simulink model "Libreria"  (R2017a)
settings: Solver=VariableStepAuto  StartTime=0.0  StopTime=10.0  RelTol=1e-3
undefined symbols (not defined in the file or in its folder): st_time3
libraries: fl_lib x63, powerlib x30, nesl_utility x24, powerlib_meascontrol x9
(part 1 of 2)
settings Model: Creator=erich  LastModifiedBy=erich

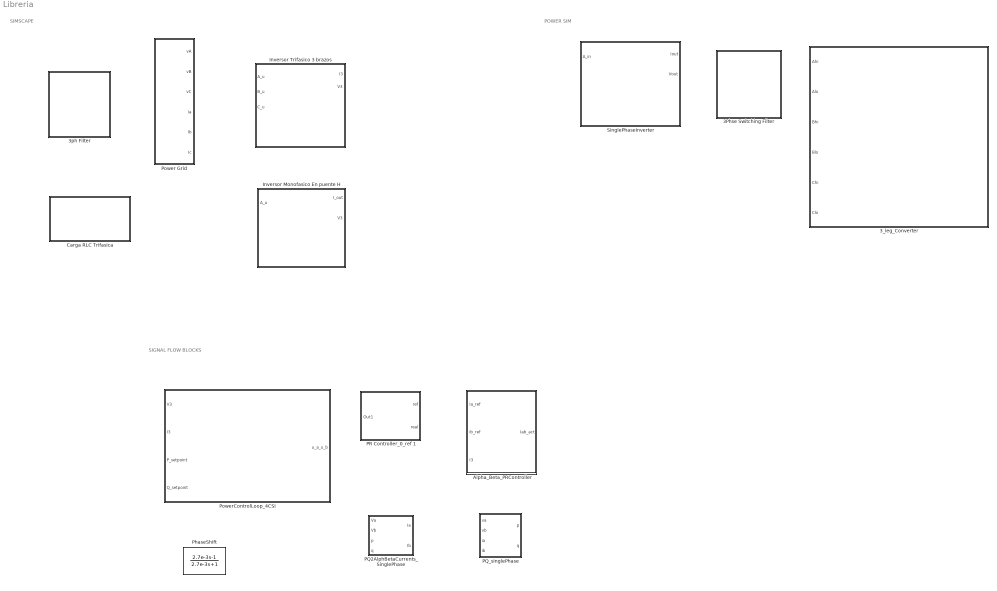
== system Libreria ==
  note: SIMSCAPE
  note: POWER SIM
  note: SIGNAL FLOW BLOCKS
  3Phse Switching Filter : Subsystem  mask{Lf=4e-3, rLf=1e-3, Cf=2.2e-6, rCf=1e-3}
      mask prompts: Lf "Inductancia (H)"; rLf "Resistencia parasita serie L (Ohm)"; Cf "Capacitancia (f)"; rCf "Resistencia parasita C serie"
      mask DialogControl DescTextVar Prompt: Configuracion del Filtro LC
      mask Display:
      | port_label('lconn', 1, 'A_{in}', 'texmode', 'on')
      | port_label('lconn', 2, 'B_{in}', 'texmode', 'on')
      | port_label('lconn', 3, 'B_{in}', 'texmode', 'on')
      | port_label('rconn', 1, 'A_{out}', 'texmode', 'on')
      | port_label('rconn', 2, 'B_{out}', 'texmode', 'on')
      | port_label('rconn', 3, 'C_{out}', 'texmode', 'on')
      | 
      | 
      | plot([.2 .5], [.7 .7])
      | plot([.5 .6], [.7 .3])
      | plot([.6 .7], [.3 .3])
      | 
      | text(.2, .8, '\fontsize{12} H(\omega)', 'texmode', 'on')
      | text(.6, .25, '\fontsize{12} \omega', 'texmode', 'on')
  3_leg_Converter : Subsystem
      mask Display:
      | port_label('input', 1, 'Ahi')
      | port_label('input', 2, 'Alo')
      | port_label('input', 3, 'Bhi')
      | port_label('input', 4, 'Blo')
      | port_label('input', 5, 'Chi')
      | port_label('input', 6, 'Clo')
      | 
      | port_label('rconn', 1, 'A')
      | port_label('rconn', 2, 'B')
      | port_label('rconn', 3, 'C')
      | port_label('rconn', 4, 'Collector')
      | port_label('rconn', 5, 'Emitter')
      | 
      | lvx = [.1 .1];
      | lvy = [.1 .2];
      | lhx = [.1 .2];
      | lhy = [.1 .1];
      | 
      | 
      | % se dibujan los interruptores de la izquierda
      | plot(lvx+.07, lvy*.8+.028+.1)
      | plot(lvx+.1, lvy+.1)
      | plot(lhx*.5+.15, lhy+.1)
      | plot(lhx*.5+.15, lhy+.2)
      | plot(lhx*.5+.07, lhy+.15)
      | 
      | d=0.5;
      | 
      | plot(lvx+.07, lvy*.8+.028+.1+d)
      | plot(lvx+.1, lvy+.1+d)
      | plot(lhx*.5+.15, lhy+.1+d)
      | plot(lhx*.5+.15, lhy+.2+d)
      | plot(lhx*.5+.07, lhy+.15+d)
      | 
      | 
      | % se dibujan los interruptores del medio
      | h=.3;
      | 
      | plot(lvx+.07+h, lvy*.8+.028+.1)
      | plot(lvx+.1+h, lvy+.1)
      | plot(lhx*.5+.15+h, lhy+.1)
      | plot(lhx*.5+.15+h, lhy+.2)
      | plot(lhx*.5+.07+h, lhy+.15)
      | 
      | plot(lvx+.07+h, lvy*.8+.028+.1+d)
      | plot(lvx+.1+h, lvy+.1+d)
      | plot(lhx*.5+.15+h, lhy+.1+d)
      | plot(lhx*.5+.15+h, lhy+.2+d)
      | plot(lhx*.5+.07+h, lhy+.15+d)
      | 
      | % se dibujan los interruptores de la derecha
      | h=.6
      | 
      | plot(lvx+.07+h, lvy*.8+.028+.1)
      | plot(lvx+.1+h, lvy+.1)
      | plot(lhx*.5+.15+h, lhy+.1)
      | plot(lhx*.5+.15+h, lhy+.2)
      | plot(lhx*.5+.07+h, lhy+.15)
      | 
      | plot(lvx+.07+h, lvy*.8+.028+.1+d)
      | plot(lvx+.1+h, lvy+.1+d)
      | plot(lhx*.5+.15+h, lhy+.1+d)
      | plot(lhx*.5+.15+h, lhy+.2+d)
      | plot(lhx*.5+.07+h, lhy+.15+d)
      | 
      | 
      | % se conectan los interruptores.
      | plot(lvx+.15, lvy*4-.1)
      | plot(lvx+.15+.3, lvy*4-.1)
      | plot(lvx+.15+.6, lvy*4-.1)
      | 
      | 
      | plot(lvx+.15, lvy+.7)
      | plot(lvx+.15+.3, lvy+.7)
      | plot(lvx+.15+.6, lvy+.7)
      | 
      | plot(lvx+.15, lvy)
      | plot(lvx+.15+.3, lvy)
      | plot(lvx+.15+.6, lvy)
      | 
      | plot(lhx*6-.35, lhy)
      | plot(lhx*6-.35, lhy+.8)
      | 
      | % raul esteban alzate 313 515 86 11
  3ph Filter : Subsystem
  Alpha_Beta_PRController : Subsystem
      mask Display:
      | port_label('input', 1, '\fontsize{13} \alpha_{ref}', 'texmode', 'on')
      | port_label('input', 2, '\fontsize{13} \beta_{ref}', 'texmode', 'on')
      | port_label('input', 3, '\fontsize{13} [ a, b, c ]', 'texmode', 'on')
      | 
      | port_label('output', 1, '\fontsize{13} [ u_{a}, u_{b}, u_{c} ]', 'texmode', 'on')
      | 
      | 
      | %plot([.4 .6],.05+[.5 .7])
      | %plot([.4 .6],.05+[.9 .7])
      | %plot([.4 .4],.05+[.9 .5])
      | 
      | text(.53,.2,'\fontsize{25} \int', 'texmode', 'on')
      | plot(.65+[0:.01:pi/10], .2+sin(40*[0:.01:pi/10])/13)
      | 
      | %text(.5,.8,'\fontsize{15} PR_{\alpha \beta}', 'texmode', 'on')
  Carga RLC Trifasica : Subsystem
      mask Display:
      | port_label('lconn', 1, 'GND')
      | 
      | port_label('rconn', 1, 'Z_1', 'texmode', 'on')
      | port_label('rconn', 2, 'Z_2', 'texmode', 'on')
      | port_label('rconn', 3, 'Z_3', 'texmode', 'on')
      | 
      | plot([.15 .25], [.4 .4])
      | plot([.15 .25], [.48 .48])
      | plot([.20 .20], [.48 .6])
      | plot([.20 .20], [.4 .28])
      | 
      | plot(.43+abs(sin(200*[.2:.001:.5]/(2*pi))/15), [.2:.001:.5]+.1)
      | plot([.438 .438], [.2 .3])
      | plot([.438 .438], [.6 .7])
      | 
      | 
      | plot([.67 .73], [.6 .6])
      | plot([.67 .73], [.3 .3])
      | 
      | plot([.7 .7], [.2 .3])
      | plot([.7 .7], [.6 .7])
      | 
      | plot([.67 .67], [.6 .3])
      | plot([.73 .73], [.6 .3])
  Inversor Monofasico En puente H : Subsystem
      mask Display:
      | port_label('input', 1, 'Mos IN')
      | 
      | port_label('lconn', 1, 'DC +')
      | port_label('lconn', 2, 'DC -')
      | 
      | 
      | port_label('rconn', 1, 'out +')
      | port_label('rconn', 2, 'out -')
      | 
      | 
      | port_label('output', 1, 'I_{out}', 'texmode', 'on')
      | port_label('output', 2, 'V_{out}', 'texmode', 'on')
      | 
      | plot([0.1 .9], [0.1 .9])
      | plot([0.2 .4], [.7 .7])
      | plot([0.2 .24], [.65 .65])
      | plot([0.28 .32], [.65 .65])
      | plot([0.36 .40], [.65 .65])
      | 
      | plot([.5:.01:.7], .25+sin(30*[.2:.01:.4])/10)
  Inversor Trifasico 3 brazos : Subsystem
      mask Display:
      | port_label('input', 1, 'A_u')
      | port_label('input', 2, 'B_u')
      | port_label('input', 3, 'C_u')
      | 
      | port_label('lconn', 1, 'DC +')
      | port_label('lconn', 2, 'DC -')
      | 
      | 
      | port_label('rconn', 1, 'A')
      | port_label('rconn', 2, 'B')
      | port_label('rconn', 3, 'C')
      | 
      | port_label('output', 1, 'I_{3\Phi}', 'texmode', 'on')
      | port_label('output', 2, 'V_{3\Phi}', 'texmode', 'on')
      | 
      | plot([0.1 .9], [0.1 .9])
      | plot([0.2 .4], [.7 .7])
      | plot([0.2 .24], [.65 .65])
      | plot([0.28 .32], [.65 .65])
      | plot([0.36 .40], [.65 .65])
      | 
      | plot([.5:.01:.7], .25+sin(30*[.2:.01:.4])/10)
  PQ2AlphBetaCurrents_SinglePhase : MATLAB Function  TreatAsAtomicUnit=on
  PQ_singlePhase : MATLAB Function  TreatAsAtomicUnit=on
  PR Controller_0_ref 1 : Subsystem  mask{Kp=2/100, Ki=10, wa=20, w0=60*2*pi, st_time=2e-3}
      mask prompts: Kp "Ganancia Proporcional"; Ki "Ganancia Integral"; wa "Ancho camapana resonancia"; w0 "Frecuencia Central"; st_time "Tiempo muerto (Start)"
      mask Display:
      | port_label('input',1,'ref')
      | port_label('input',2,'sens')
      | port_label('output',1,'out')
      | 
      | plot(.4+[0:.01:pi/10], .32+sin(40*[0:.01:pi/10])/13)
      | 
      | plot([.4 .6],.05+[.5 .7])
      | plot([.4 .6],.05+[.9 .7])
      | plot([.4 .4],.05+[.9 .5])
      | 
      | text(.27,.37,'\fontsize{25} \int', 'texmode', 'on')
  PhaseShift : TransferFcn  Numerator=[2.7e-3 -1]  Denominator=[2.7e-3 1]
  Power Grid : Subsystem
  PowerControlLoop_4CSI : Subsystem
      mask Display:
      | port_label('input', 1, '\fontsize{14} V_{abc}', 'texmode', 'on')
      | port_label('input', 2, '\fontsize{14} I_{abc}', 'texmode', 'on')
      | port_label('input', 3, '\fontsize{14} P_{set}', 'texmode', 'on')
      | port_label('input', 4, '\fontsize{14} Q_{set}', 'texmode', 'on')
      | port_label('output', 1, '\fontsize{14} u_{\alpha, \beta}', 'texmode', 'on')
      | 
      | 
      | disp('\fontsize{12} Power Control for 3\Phi CSI', 'texmode', 'on')
  SinglePhaseInverter : Subsystem  mask{st_time=2e-3, f_sw=10000}
      mask prompts: st_time "Tiempo muerto (Start)"; f_sw "Switching frequency"
      mask Display:
      | port_label('input', 1, 'd', 'texmode', 'on')
      | 
      | port_label('lconn', 1, 'DC +')
      | port_label('lconn', 2, 'DC -')
      | 
      | 
      | port_label('rconn', 1, 'V_{out+}')
      | port_label('rconn', 2, 'B_{out-}')
      | 
      | 
      | port_label('output', 1, 'I_{out}', 'texmode', 'on')
      | port_label('output', 2, 'V_{out}', 'texmode', 'on')
      | 
      | plot([0.1 .9], [0.1 .9])
      | plot([0.2 .4], [.7 .7])
      | plot([0.2 .24], [.65 .65])
      | plot([0.28 .32], [.65 .65])
      | plot([0.36 .40], [.65 .65])
      | 
      | plot([.5:.01:.7], .25+sin(30*[.2:.01:.4])/10)

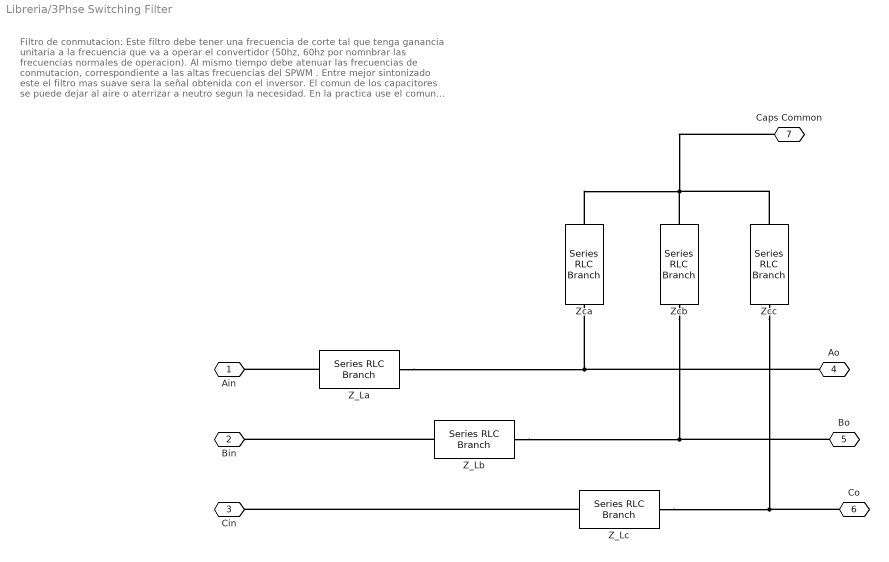
== system Libreria/3Phse Switching Filter ==
  note: Filtro de conmutacion:
      | Este filtro debe tener una frecuencia de corte tal
      | que tenga ganancia unitaria a la frecuencia que va
      | a operar el convertidor (50hz, 60hz por nomnbrar
      | las frecuencias normales de operacion). Al mismo
      | tiempo debe atenuar las frecuencias de conmutacion,
      | correspondiente a las altas frecuencias del SPWM .
      | Entre mejor sintonizado este el filtro mas suave sera
      | la señal obtenida con el inversor. El comun de los
      | capacitores se puede dejar al aire o aterrizar a neutro
      | segun la necesidad. En la practica use el comun al
      | aire para un inversor trifasico de verdad y dio buenos
      | resultados.
  Z_La : powerlib/Elements/Series RLC Branch  LConnTagsString=__new0  RConnTagsString=__new0  BranchType=RL  Resistance=rLf  Inductance=Lf  SetiL0=off  InitialCurrent=0  Capacitance=2.2e-6  Setx0=off  InitialVoltage=0  Measurements=None
  Z_Lb : powerlib/Elements/Series RLC Branch  LConnTagsString=__new0  RConnTagsString=__new0  BranchType=RL  Resistance=rLf  Inductance=Lf  SetiL0=off  InitialCurrent=0  Capacitance=2.2e-6  Setx0=off  InitialVoltage=0  Measurements=None
  Z_Lc : powerlib/Elements/Series RLC Branch  LConnTagsString=__new0  RConnTagsString=__new0  BranchType=RL  Resistance=rLf  Inductance=Lf  SetiL0=off  InitialCurrent=0  Capacitance=2.2e-6  Setx0=off  InitialVoltage=0  Measurements=None
  Zca : powerlib/Elements/Series RLC Branch  LConnTagsString=__new0  RConnTagsString=__new0  BranchType=RC  Resistance=rCf  Inductance=1e-9  SetiL0=off  InitialCurrent=0  Capacitance=Cf  Setx0=off  InitialVoltage=0  Measurements=None
  Zcb : powerlib/Elements/Series RLC Branch  LConnTagsString=__new0  RConnTagsString=__new0  BranchType=RC  Resistance=rCf  Inductance=1e-9  SetiL0=off  InitialCurrent=0  Capacitance=Cf  Setx0=off  InitialVoltage=0  Measurements=None
  Zcc : powerlib/Elements/Series RLC Branch  LConnTagsString=__new0  RConnTagsString=__new0  BranchType=RC  Resistance=rCf  Inductance=1e-9  SetiL0=off  InitialCurrent=0  Capacitance=Cf  Setx0=off  InitialVoltage=0  Measurements=None
  Ain : PMIOPort  Port=1  Side=Left
  Bin : PMIOPort  Port=2  Side=Left
  Cin : PMIOPort  Port=3  Side=Left
  Ao : PMIOPort  Port=4  Side=Right
  Bo : PMIOPort  Port=5  Side=Right
  Co : PMIOPort  Port=6  Side=Right
  Caps Common : PMIOPort  Port=7  Side=Right
  connections:
  Zcc/RConn1 -- Zcb/RConn1 -- Zca/RConn1 -- Caps Common/RConn1
  Z_Lb/RConn1 -- Bo/RConn1 -- Zcb/LConn1
  Z_Lc/RConn1 -- Co/RConn1 -- Zcc/LConn1
  Ao/RConn1 -- Z_La/RConn1 -- Zca/LConn1
  Z_La/LConn1 -- Ain/RConn1
  Z_Lb/LConn1 -- Bin/RConn1
  Z_Lc/LConn1 -- Cin/RConn1

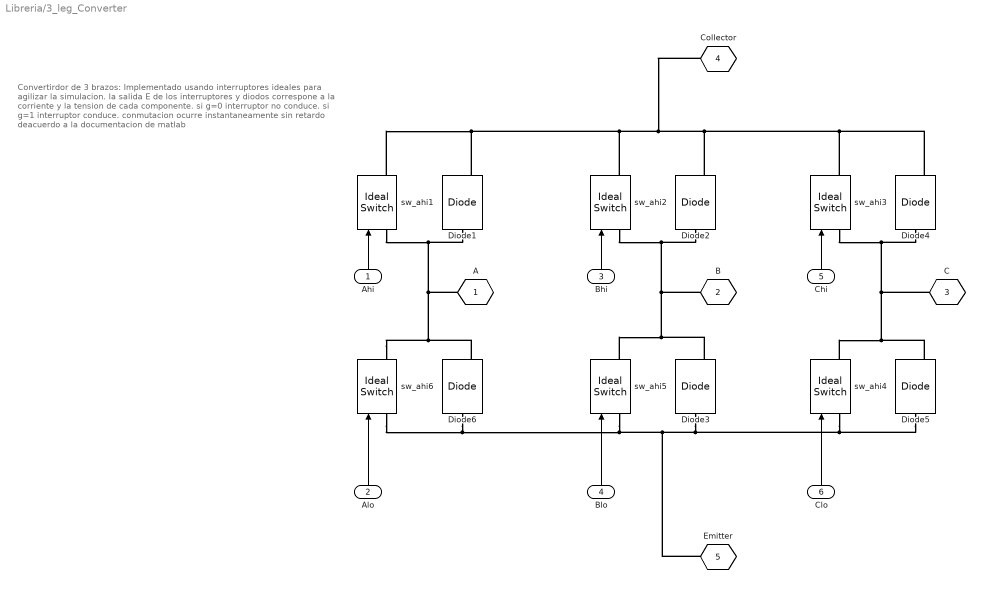
== system Libreria/3_leg_Converter ==
  note: Convertirdor de 3 brazos:
      |
      | Implementado usando interruptores
      | ideales para agilizar la simulacion.
      | la salida E de los interruptores y diodos correspone
      | a la corriente y la tension de cada componente.
      |
      | si g=0 interruptor no conduce.
      | si g=1 interruptor conduce.
      |
      | conmutacion ocurre instantaneamente sin
      | retardo deacuerdo a la documentacion de matlab
  Ahi : Inport
  Alo : Inport  Port=2
  Bhi : Inport  Port=3
  Blo : Inport  Port=4
  Chi : Inport  Port=5
  Clo : Inport  Port=6
   sw_ahi{1..6} (6 alike) : powerlib/Power Electronics/Ideal Switch  Ron=20e-3  Lon=0  IC=0  Rs=1e6  Cs=10e-12  Measurements=on
  Diode{1..6} (6 alike) : powerlib/Power Electronics/Diode  Ron=.2  Lon=0  Vf=0.8  IC=0  UseSnubber=0  Rs=0  Cs=0  Measurements=on
  " A" : PMIOPort  Tag=PMCPort  Port=1  Side=Right
  B : PMIOPort  Tag=PMCPort  Port=2  Side=Right
  C : PMIOPort  Tag=PMCPort  Port=3  Side=Right
  Collector : PMIOPort  Tag=PMCPort  Port=4  Side=Right
  Emitter : PMIOPort  Tag=PMCPort  Port=5  Side=Right
  wires:
  Clo/1 -> " sw_ahi4"/1
  Alo/1 -> " sw_ahi6"/1
  Ahi/1 -> " sw_ahi1"/1
  Blo/1 -> " sw_ahi5"/1
  Bhi/1 -> " sw_ahi2"/1
  Chi/1 -> " sw_ahi3"/1
  connections:
  Diode3/RConn1 -- " sw_ahi5"/RConn1 -- B/RConn1 -- " sw_ahi2"/LConn1 -- Diode2/LConn1
  Diode3/LConn1 -- " sw_ahi4"/LConn1 -- Diode5/LConn1 -- Emitter/RConn1 -- " sw_ahi5"/LConn1 -- Diode6/LConn1 -- " sw_ahi6"/LConn1
  Diode2/RConn1 -- " sw_ahi3"/RConn1 -- Diode4/RConn1 -- Collector/RConn1 -- " sw_ahi2"/RConn1 -- " sw_ahi1"/RConn1 -- Diode1/RConn1
  " sw_ahi6"/RConn1 -- Diode6/RConn1 -- " A"/RConn1 -- " sw_ahi1"/LConn1 -- Diode1/LConn1
  " sw_ahi4"/RConn1 -- Diode5/RConn1 -- C/RConn1 -- " sw_ahi3"/LConn1 -- Diode4/LConn1

== system Libreria/3ph Filter ==
  CdcS1 : fl_lib/Electrical/Electrical Elements/Capacitor  c=3.5 uF  r=1e-6 Ohm  g=0 1/Ohm  i_specify=off  i_priority=None  i=0 A  i_nominal_specify=off  i_nominal_unit=A  i_nominal_value=1  v_specify=off  v_priority=None  v=0 V  v_nominal_specify=off  v_nominal_unit=V  v_nominal_value=1  vc_specify=on  vc_priority=High  vc=0 V  vc_nominal_specify=off  vc_nominal_unit=V  vc_nominal_value=1
  CdcS2 : fl_lib/Electrical/Electrical Elements/Capacitor  c=3.5 uF  r=1e-6 Ohm  g=0 1/Ohm  i_specify=off  i_priority=None  i=0 A  i_nominal_specify=off  i_nominal_unit=A  i_nominal_value=1  v_specify=off  v_priority=None  v=0 V  v_nominal_specify=off  v_nominal_unit=V  v_nominal_value=1  vc_specify=on  vc_priority=High  vc=0 V  vc_nominal_specify=off  vc_nominal_unit=V  vc_nominal_value=1
  CdcS3 : fl_lib/Electrical/Electrical Elements/Capacitor  c=3.5 uF  r=1e-6 Ohm  g=0 1/Ohm  i_specify=off  i_priority=None  i=0 A  i_nominal_specify=off  i_nominal_unit=A  i_nominal_value=1  v_specify=off  v_priority=None  v=0 V  v_nominal_specify=off  v_nominal_unit=V  v_nominal_value=1  vc_specify=on  vc_priority=High  vc=0 V  vc_nominal_specify=off  vc_nominal_unit=V  vc_nominal_value=1
  LA_filt : fl_lib/Electrical/Electrical Elements/Inductor  l=6.2 mH  r=0.1 Ohm  g=1e-6 1/Ohm  i_specify=off  i_priority=None  i=0 A  i_nominal_specify=off  i_nominal_unit=A  i_nominal_value=1  v_specify=off  v_priority=None  v=0 V  v_nominal_specify=off  v_nominal_unit=V  v_nominal_value=1  i_L_specify=on  i_L_priority=High  i_L=0 A  i_L_nominal_specify=off  i_L_nominal_unit=A  i_L_nominal_value=1
  LB_filt : fl_lib/Electrical/Electrical Elements/Inductor  l=6.2 mH  r=2 Ohm  g=1e-6 1/Ohm  i_specify=off  i_priority=None  i=0 A  i_nominal_specify=off  i_nominal_unit=A  i_nominal_value=1  v_specify=off  v_priority=None  v=0 V  v_nominal_specify=off  v_nominal_unit=V  v_nominal_value=1  i_L_specify=on  i_L_priority=High  i_L=0 A  i_L_nominal_specify=off  i_L_nominal_unit=A  i_L_nominal_value=1
  LC_filt : fl_lib/Electrical/Electrical Elements/Inductor  l=6.2 mH  r=2 Ohm  g=1e-6 1/Ohm  i_specify=off  i_priority=None  i=0 A  i_nominal_specify=off  i_nominal_unit=A  i_nominal_value=1  v_specify=off  v_priority=None  v=0 V  v_nominal_specify=off  v_nominal_unit=V  v_nominal_value=1  i_L_specify=on  i_L_priority=High  i_L=0 A  i_L_nominal_specify=off  i_L_nominal_unit=A  i_L_nominal_value=1
  Ain : PMIOPort  Port=1  Side=Left
  Aout : PMIOPort  Port=2  Side=Right
  Bin : PMIOPort  Port=3  Side=Left
  Bout : PMIOPort  Port=4  Side=Right
  Cin : PMIOPort  Port=5  Side=Left
  Cout : PMIOPort  Port=6  Side=Right
  connections:
  CdcS1/RConn1 -- Aout/RConn1 -- LA_filt/RConn1
  CdcS2/LConn1 -- CdcS1/LConn1 -- CdcS3/LConn1
  CdcS3/RConn1 -- Bout/RConn1 -- LB_filt/RConn1
  CdcS2/RConn1 -- Cout/RConn1 -- LC_filt/RConn1
  LC_filt/LConn1 -- Cin/RConn1
  LA_filt/LConn1 -- Ain/RConn1
  LB_filt/LConn1 -- Bin/RConn1

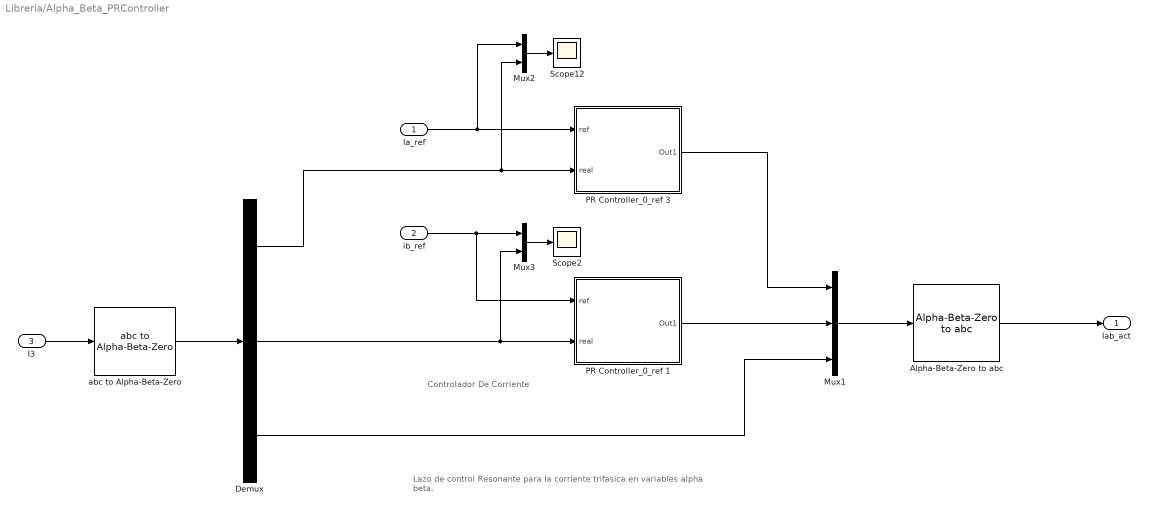
== system Libreria/Alpha_Beta_PRController ==
  note: Controlador De Corriente
  note: Lazo de control Resonante para la
      | corriente trifasica en variables alpha beta.
  Ia_ref : Inport
  ib_ref : Inport  Port=2
  I3 : Inport  Port=3
  Alpha-Beta-Zero to abc : powerlib_meascontrol/Transformations/Alpha-Beta-Zero to abc
      settings: SourceProductName=Simscape Power Systems  SourceProductBaseCode=PS
  Demux : Demux  Outputs=3
  Mux1 : Mux  Inputs=3
  Mux2 : Mux  Inputs=2
  Mux3 : Mux  Inputs=2
  PR Controller_0_ref 1 : Subsystem
      mask Display:
      | port_label('input',1,'ref')
      | port_label('input',2,'sens')
      | port_label('output',1,'out')
      | 
      | plot(.4+[0:.01:pi/10], .32+sin(40*[0:.01:pi/10])/13)
      | 
      | plot([.4 .6],.05+[.5 .7])
      | plot([.4 .6],.05+[.9 .7])
      | plot([.4 .4],.05+[.9 .5])
      | 
      | text(.27,.37,'\fontsize{25} \int', 'texmode', 'on')
  PR Controller_0_ref 3 : Subsystem
      mask Display:
      | port_label('input',1,'ref')
      | port_label('input',2,'sens')
      | port_label('output',1,'out')
      | 
      | plot(.4+[0:.01:pi/10], .32+sin(40*[0:.01:pi/10])/13)
      | 
      | plot([.4 .6],.05+[.5 .7])
      | plot([.4 .6],.05+[.9 .7])
      | plot([.4 .4],.05+[.9 .5])
      | 
      | text(.27,.37,'\fontsize{25} \int', 'texmode', 'on')
  Scope12 : Scope
  Scope2 : Scope
  abc to Alpha-Beta-Zero : powerlib_meascontrol/Transformations/abc to Alpha-Beta-Zero
      settings: SourceProductName=Simscape Power Systems
  Iab_act : Outport
  wires:
  I3/1 -> abc to Alpha-Beta-Zero/1
  Mux2/1 -> Scope12/1
  Demux/2 -> PR Controller_0_ref 1/2(real), Mux3/2
  PR Controller_0_ref 1/1(Out1) -> Mux1/2
  Mux1/1 -> Alpha-Beta-Zero to abc/1
  Mux3/1 -> Scope2/1
  Alpha-Beta-Zero to abc/1 -> Iab_act/1
  abc to Alpha-Beta-Zero/1 -> Demux/1
  ib_ref/1 -> PR Controller_0_ref 1/1(ref), Mux3/1
  Ia_ref/1 -> Mux2/1, PR Controller_0_ref 3/1(ref)
  PR Controller_0_ref 3/1(Out1) -> Mux1/1
  Demux/3 -> Mux1/3
  Demux/1 -> Mux2/2, PR Controller_0_ref 3/2(real)

== system Libreria/Carga RLC Trifasica ==
  Capacitor : fl_lib/Electrical/Electrical Elements/Capacitor  c=100e-6 uF  r=1e-6 Ohm  g=0 1/Ohm  i_specify=off  i_priority=None  i=0 A  i_nominal_specify=off  i_nominal_unit=A  i_nominal_value=1  v_specify=off  v_priority=None  v=0 V  v_nominal_specify=off  v_nominal_unit=V  v_nominal_value=1  vc_specify=off  vc_priority=High  vc=0 V  vc_nominal_specify=off  vc_nominal_unit=V  vc_nominal_value=1
  Capacitor1 : fl_lib/Electrical/Electrical Elements/Capacitor  c=100e-6 uF  r=1e-6 Ohm  g=0 1/Ohm  i_specify=off  i_priority=None  i=0 A  i_nominal_specify=off  i_nominal_unit=A  i_nominal_value=1  v_specify=off  v_priority=None  v=0 V  v_nominal_specify=off  v_nominal_unit=V  v_nominal_value=1  vc_specify=off  vc_priority=High  vc=0 V  vc_nominal_specify=off  vc_nominal_unit=V  vc_nominal_value=1
  Capacitor2 : fl_lib/Electrical/Electrical Elements/Capacitor  c=100e-6 uF  r=1e-6 Ohm  g=0 1/Ohm  i_specify=off  i_priority=None  i=0 A  i_nominal_specify=off  i_nominal_unit=A  i_nominal_value=1  v_specify=off  v_priority=None  v=0 V  v_nominal_specify=off  v_nominal_unit=V  v_nominal_value=1  vc_specify=off  vc_priority=High  vc=0 V  vc_nominal_specify=off  vc_nominal_unit=V  vc_nominal_value=1
  Inductor : fl_lib/Electrical/Electrical Elements/Inductor  l=5200 mH  r=0 Ohm  g=100e-9 1/Ohm  i_specify=off  i_priority=None  i=0 A  i_nominal_specify=off  i_nominal_unit=A  i_nominal_value=1  v_specify=off  v_priority=None  v=0 V  v_nominal_specify=off  v_nominal_unit=V  v_nominal_value=1  i_L_specify=off  i_L_priority=High  i_L=0 A  i_L_nominal_specify=off  i_L_nominal_unit=A  i_L_nominal_value=1
  Inductor1 : fl_lib/Electrical/Electrical Elements/Inductor  l=5200 mH  r=0 Ohm  g=100e-9 1/Ohm  i_specify=off  i_priority=None  i=0 A  i_nominal_specify=off  i_nominal_unit=A  i_nominal_value=1  v_specify=off  v_priority=None  v=0 V  v_nominal_specify=off  v_nominal_unit=V  v_nominal_value=1  i_L_specify=off  i_L_priority=High  i_L=0 A  i_L_nominal_specify=off  i_L_nominal_unit=A  i_L_nominal_value=1
  Inductor2 : fl_lib/Electrical/Electrical Elements/Inductor  l=5200 mH  r=0 Ohm  g=100e-9 1/Ohm  i_specify=off  i_priority=None  i=0 A  i_nominal_specify=off  i_nominal_unit=A  i_nominal_value=1  v_specify=off  v_priority=None  v=0 V  v_nominal_specify=off  v_nominal_unit=V  v_nominal_value=1  i_L_specify=off  i_L_priority=High  i_L=0 A  i_L_nominal_specify=off  i_L_nominal_unit=A  i_L_nominal_value=1
  RLA : fl_lib/Electrical/Electrical Elements/Resistor  R=15 Ohm  i_specify=off  i_priority=None  i=0 A  i_nominal_specify=off  i_nominal_unit=A  i_nominal_value=1  v_specify=off  v_priority=None  v=0 V  v_nominal_specify=off  v_nominal_unit=V  v_nominal_value=1
  RLB : fl_lib/Electrical/Electrical Elements/Resistor  R=15 Ohm  i_specify=off  i_priority=None  i=0 A  i_nominal_specify=off  i_nominal_unit=A  i_nominal_value=1  v_specify=off  v_priority=None  v=0 V  v_nominal_specify=off  v_nominal_unit=V  v_nominal_value=1
  RLC : fl_lib/Electrical/Electrical Elements/Resistor  R=15 Ohm  i_specify=off  i_priority=None  i=0 A  i_nominal_specify=off  i_nominal_unit=A  i_nominal_value=1  v_specify=off  v_priority=None  v=0 V  v_nominal_specify=off  v_nominal_unit=V  v_nominal_value=1
  Conn1 : PMIOPort  Port=1  Side=Right
  Conn2 : PMIOPort  Port=2  Side=Right
  Conn3 : PMIOPort  Port=3  Side=Right
  Conn4 : PMIOPort  Port=4  Side=Left
  connections:
  RLB/RConn1 -- Capacitor1/RConn1 -- Inductor1/RConn1 -- Conn4/RConn1 -- Inductor2/RConn1 -- Capacitor/RConn1 -- RLA/RConn1 -- Capacitor2/RConn1 -- Inductor/RConn1 -- RLC/RConn1
  RLA/LConn1 -- Inductor2/LConn1 -- Conn1/RConn1 -- Capacitor/LConn1
  RLC/LConn1 -- Capacitor2/LConn1 -- Conn3/RConn1 -- Inductor/LConn1
  RLB/LConn1 -- Conn2/RConn1 -- Capacitor1/LConn1 -- Inductor1/LConn1

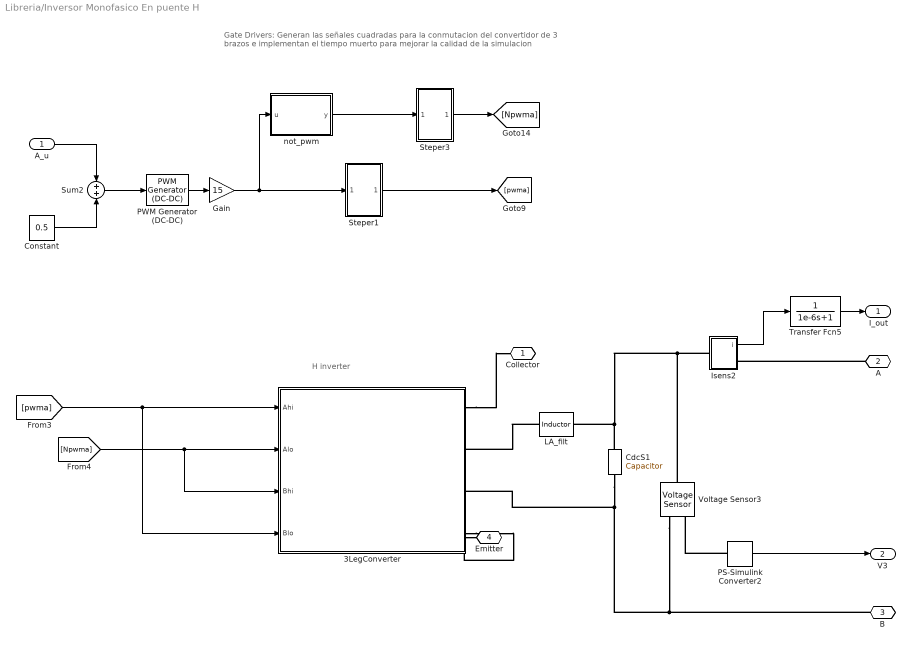
== system Libreria/Inversor Monofasico En puente H ==
  note: Gate Drivers: Generan las señales cuadradas para
      | la conmutacion del convertidor de 3 brazos e implementan el
      | tiempo muerto para mejorar la calidad de la simulacion
  note: H inverter
  A_u : Inport
  3LegConverter : Subsystem
      mask Display:
      | % entradas de conmutacion del mosfet
      | port_label('input',1,'Ahi')
      | port_label('input',2,'Alo')
      | port_label('input',3,'Bhi')
      | port_label('input',4,'Blo')
      | 
      | 
      | % puertos de conexion del inversor
      | port_label('rconn',1,'Collector') % + fuente dc
      | port_label('rconn',2,'Out +') % fase A
      | port_label('rconn',3,'Out -') % fase B
      | port_label('rconn',4,'Emitter') % ref fuente dc
      | 
      | 
      | plot([.4 .4],[.35 .7])
      | plot([.2 .4],[.52 .52])
      | plot([.46 .46],[.22 .85])
      | plot([.46 .7],[.73 .73])
      | plot([.46 .7],[.32 .32])
  CdcS1 : fl_lib/Electrical/Electrical Elements/Capacitor  c=3.5 uF  r=1e-6 Ohm  g=0 1/Ohm  i_specify=off  i_priority=None  i=0 A  i_nominal_specify=off  i_nominal_unit=A  i_nominal_value=1  v_specify=off  v_priority=None  v=0 V  v_nominal_specify=off  v_nominal_unit=V  v_nominal_value=1  vc_specify=on  vc_priority=High  vc=0 V  vc_nominal_specify=off  vc_nominal_unit=V  vc_nominal_value=1
  Constant : Constant  Value=0.5
  Gain : Gain  Gain=15
  Isens2 : Subsystem
  LA_filt : fl_lib/Electrical/Electrical Elements/Inductor  l=6.2 mH  r=0.1 Ohm  g=1e-6 1/Ohm  i_specify=off  i_priority=None  i=0 A  i_nominal_specify=off  i_nominal_unit=A  i_nominal_value=1  v_specify=off  v_priority=None  v=0 V  v_nominal_specify=off  v_nominal_unit=V  v_nominal_value=1  i_L_specify=on  i_L_priority=High  i_L=0 A  i_L_nominal_specify=off  i_L_nominal_unit=A  i_L_nominal_value=1
  PS-Simulink Converter2 : nesl_utility/PS-Simulink Converter  PhysicalDomain=network_engine_domain  SubClassName=ps_output  LeftPortType=input  RightPortType=output  PseudoPeriodic=off  Frequencies=[]  Unit=1  AffineConversion=off
  PWM Generator (DC-DC) : powerlib_meascontrol/Pulse & Signal Generators/PWM Generator (DC-DC)  Fsw=5000  Ts=0
  Steper1 : Subsystem
  Steper3 : Subsystem
  Sum2 : Sum
  Transfer Fcn5 : TransferFcn  Denominator=[1e-6 1]
  Voltage Sensor3 : fl_lib/Electrical/Electrical Sensors/Voltage Sensor
  not_pwm : MATLAB Function  TreatAsAtomicUnit=on
  Collector : PMIOPort  Port=1  Side=Left
  A : PMIOPort  Port=2  Side=Right
  B : PMIOPort  Port=3  Side=Right
  Emitter : PMIOPort  Port=4  Side=Left
  I_out : Outport
  V3 : Outport  Port=2
  wires:
  [pwma] -> 3LegConverter/4(Blo), 3LegConverter/1(Ahi)
  [Npwma] -> 3LegConverter/3(Bhi), 3LegConverter/2(Alo)
  Gain/1 -> Steper1/1(In1), not_pwm/1(u)
  Steper3/1(Out1) -> [Npwma]
  Constant/1 -> Sum2/2
  Sum2/1 -> PWM Generator (DC-DC)/1
  not_pwm/1(y) -> Steper3/1(In1)
  PWM Generator (DC-DC)/1 -> Gain/1
  Steper1/1(Out1) -> [pwma]
  A_u/1 -> Sum2/1
  Isens2/1(i) -> Transfer Fcn5/1
  PS-Simulink Converter2/1 -> V3/1
  Transfer Fcn5/1 -> I_out/1
  connections:
  3LegConverter/RConn4 -- Emitter/RConn1
  3LegConverter/RConn1 -- Collector/RConn1
  A/RConn1 -- Isens2/RConn1
  PS-Simulink Converter2/LConn1 -- Voltage Sensor3/RConn1
  CdcS1/RConn1 -- Isens2/LConn1 -- Voltage Sensor3/LConn1 -- LA_filt/RConn1
  LA_filt/LConn1 -- 3LegConverter/RConn2
  CdcS1/LConn1 -- B/RConn1 -- Voltage Sensor3/RConn2 -- 3LegConverter/RConn3

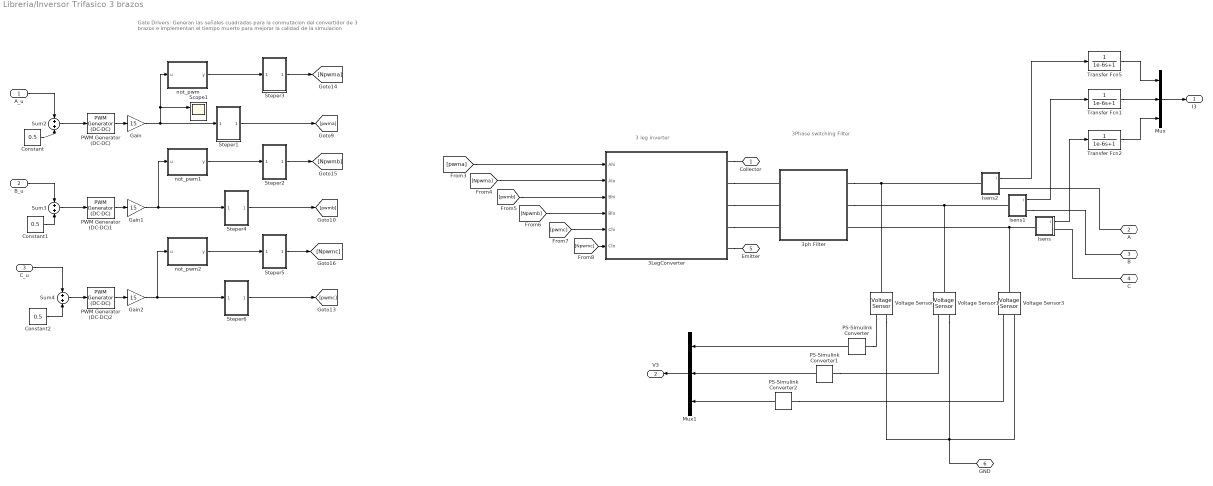
== system Libreria/Inversor Trifasico 3 brazos ==
  note: Gate Drivers: Generan las señales cuadradas para
      | la conmutacion del convertidor de 3 brazos e implementan el
      | tiempo muerto para mejorar la calidad de la simulacion
  note: 3 leg inverter
  note: 3Phase
      | switching
      | Filter
  A_u : Inport
  B_u : Inport  Port=2
  C_u : Inport  Port=3
  3LegConverter : Subsystem
      mask Display:
      | % entradas de conmutacion del mosfet
      | port_label('input',1,'Ahi')
      | port_label('input',2,'Alo')
      | port_label('input',3,'Bhi')
      | port_label('input',4,'Blo')
      | port_label('input',5,'Chi')
      | port_label('input',6,'Clo')
      | 
      | % puertos de conexion del inversor
      | port_label('rconn',1,'Collector') % + fuente dc
      | port_label('rconn',2,'A') % fase A
      | port_label('rconn',3,'B') % fase B
      | port_label('rconn',4,'C') % fase C
      | port_label('rconn',5,'Emitter') % ref fuente dc
      | 
      | 
      | plot([.4 .4],[.35 .7])
      | plot([.2 .4],[.52 .52])
      | plot([.46 .46],[.22 .85])
      | plot([.46 .7],[.73 .73])
      | plot([.46 .7],[.32 .32])
  3ph Filter : Subsystem
  Constant : Constant  Value=0.5
  Constant1 : Constant  Value=0.5
  Constant2 : Constant  Value=0.5
  Gain : Gain  Gain=15
  Gain1 : Gain  Gain=15
  Gain2 : Gain  Gain=15
  Isens : Subsystem
  Isens1 : Subsystem
  Isens2 : Subsystem
  Mux : Mux  Inputs=3
  Mux1 : Mux  Inputs=3
  PS-Simulink Converter : nesl_utility/PS-Simulink Converter  PhysicalDomain=network_engine_domain  SubClassName=ps_output  LeftPortType=input  RightPortType=output  PseudoPeriodic=off  Frequencies=[]  Unit=1  AffineConversion=off
  PS-Simulink Converter1 : nesl_utility/PS-Simulink Converter  PhysicalDomain=network_engine_domain  SubClassName=ps_output  LeftPortType=input  RightPortType=output  PseudoPeriodic=off  Frequencies=[]  Unit=1  AffineConversion=off
  PS-Simulink Converter2 : nesl_utility/PS-Simulink Converter  PhysicalDomain=network_engine_domain  SubClassName=ps_output  LeftPortType=input  RightPortType=output  PseudoPeriodic=off  Frequencies=[]  Unit=1  AffineConversion=off
  PWM Generator (DC-DC) : powerlib_meascontrol/Pulse & Signal Generators/PWM Generator (DC-DC)  Fsw=5000  Ts=0
  PWM Generator (DC-DC)1 : powerlib_meascontrol/Pulse & Signal Generators/PWM Generator (DC-DC)  Fsw=5000  Ts=0
  PWM Generator (DC-DC)2 : powerlib_meascontrol/Pulse & Signal Generators/PWM Generator (DC-DC)  Fsw=5000  Ts=0
  Scope1 : Scope  NumInputPorts=2
  Steper1 : Subsystem
  Steper2 : Subsystem
  Steper3 : Subsystem
  Steper4 : Subsystem
  Steper5 : Subsystem
  Steper6 : Subsystem
  Sum2 : Sum
  Sum3 : Sum
  Sum4 : Sum
  Transfer Fcn1 : TransferFcn  Denominator=[1e-6 1]
  Transfer Fcn2 : TransferFcn  Denominator=[1e-6 1]
  Transfer Fcn5 : TransferFcn  Denominator=[1e-6 1]
  Voltage Sensor : fl_lib/Electrical/Electrical Sensors/Voltage Sensor
  Voltage Sensor1 : fl_lib/Electrical/Electrical Sensors/Voltage Sensor
  Voltage Sensor3 : fl_lib/Electrical/Electrical Sensors/Voltage Sensor
  not_pwm : MATLAB Function  TreatAsAtomicUnit=on
  not_pwm1 : MATLAB Function  TreatAsAtomicUnit=on
  not_pwm2 : MATLAB Function  TreatAsAtomicUnit=on
  Collector : PMIOPort  Port=1  Side=Left
  A : PMIOPort  Port=2  Side=Right
  B : PMIOPort  Port=3  Side=Right
  C : PMIOPort  Port=4  Side=Right
  Emitter : PMIOPort  Port=5  Side=Left
  GND : PMIOPort  Port=6  Side=Right
  I3 : Outport
  V3 : Outport  Port=2
  wires:
  C_u/1 -> Sum4/1
  [Npwmc] -> 3LegConverter/6(Clo)
  [pwma] -> 3LegConverter/1(Ahi)
  [pwmc] -> 3LegConverter/5(Chi)
  [Npwma] -> 3LegConverter/2(Alo)
  [Npwmb] -> 3LegConverter/4(Blo)
  [pwmb] -> 3LegConverter/3(Bhi)
  Steper5/1(Out1) -> [Npwmc]
  Steper4/1(Out1) -> [pwmb]
  Gain/1 -> Steper1/1(In1), Scope1/1, not_pwm/1(u)
  not_pwm1/1(y) -> Steper2/1(In1)
  Steper3/1(Out1) -> [Npwma]
  Constant/1 -> Sum2/2
  Sum2/1 -> PWM Generator (DC-DC)/1
  Gain2/1 -> Steper6/1(In1), not_pwm2/1(u)
  Sum3/1 -> PWM Generator (DC-DC)1/1
  Steper6/1(Out1) -> [pwmc]
  Sum4/1 -> PWM Generator (DC-DC)2/1
  Gain1/1 -> Steper4/1(In1), not_pwm1/1(u)
  not_pwm2/1(y) -> Steper5/1(In1)
  Steper2/1(Out1) -> [Npwmb]
  Constant2/1 -> Sum4/2
  PWM Generator (DC-DC)1/1 -> Gain1/1
  not_pwm/1(y) -> Steper3/1(In1)
  PWM Generator (DC-DC)/1 -> Gain/1
  PWM Generator (DC-DC)2/1 -> Gain2/1
  Steper1/1(Out1) -> [pwma]
  Constant1/1 -> Sum3/2
  B_u/1 -> Sum3/1
  A_u/1 -> Sum2/1
  Isens/1(i) -> Transfer Fcn2/1
  Isens1/1(i) -> Transfer Fcn1/1
  Isens2/1(i) -> Transfer Fcn5/1
  Mux/1 -> I3/1
  Transfer Fcn1/1 -> Mux/2
  Transfer Fcn5/1 -> Mux/1
  Transfer Fcn2/1 -> Mux/3
  Mux1/1 -> V3/1
  PS-Simulink Converter/1 -> Mux1/1
  PS-Simulink Converter1/1 -> Mux1/2
  PS-Simulink Converter2/1 -> Mux1/3
  connections:
  3LegConverter/RConn5 -- Emitter/RConn1
  3LegConverter/RConn1 -- Collector/RConn1
  C/RConn1 -- Isens/RConn1
  Isens1/RConn1 -- B/RConn1
  A/RConn1 -- Isens2/RConn1
  3LegConverter/RConn2 -- 3ph Filter/LConn1
  3LegConverter/RConn3 -- 3ph Filter/LConn2
  3LegConverter/RConn4 -- 3ph Filter/LConn3
  3ph Filter/RConn1 -- Voltage Sensor/LConn1 -- Isens2/LConn1
  3ph Filter/RConn2 -- Isens1/LConn1 -- Voltage Sensor1/LConn1
  Isens/LConn1 -- Voltage Sensor3/LConn1 -- 3ph Filter/RConn3
  Voltage Sensor1/RConn2 -- Voltage Sensor3/RConn2 -- GND/RConn1 -- Voltage Sensor/RConn2
  PS-Simulink Converter1/LConn1 -- Voltage Sensor1/RConn1
  PS-Simulink Converter2/LConn1 -- Voltage Sensor3/RConn1
  PS-Simulink Converter/LConn1 -- Voltage Sensor/RConn1

== system Libreria/PR Controller_0_ref 1 ==
  ref : Inport
  real : Inport  Port=2
  K1 : Gain  Gain=Kp
  K2 : Gain  Gain=Ki
  Steper6 : Subsystem
  Sum : Sum  Inputs=+-
  Sum1 : Sum  Inputs=+|+
  Transfer Fcn : TransferFcn  Numerator=[1 0]  Denominator=[1 wa (w0)^2]
  Out1 : Outport
  wires:
  real/1 -> Sum/2
  ref/1 -> Sum/1
  Sum/1 -> Steper6/1(In1)
  K1/1 -> Sum1/1
  Transfer Fcn/1 -> Sum1/2
  K2/1 -> Transfer Fcn/1
  Steper6/1(Out1) -> K1/1, K2/1
  Sum1/1 -> Out1/1

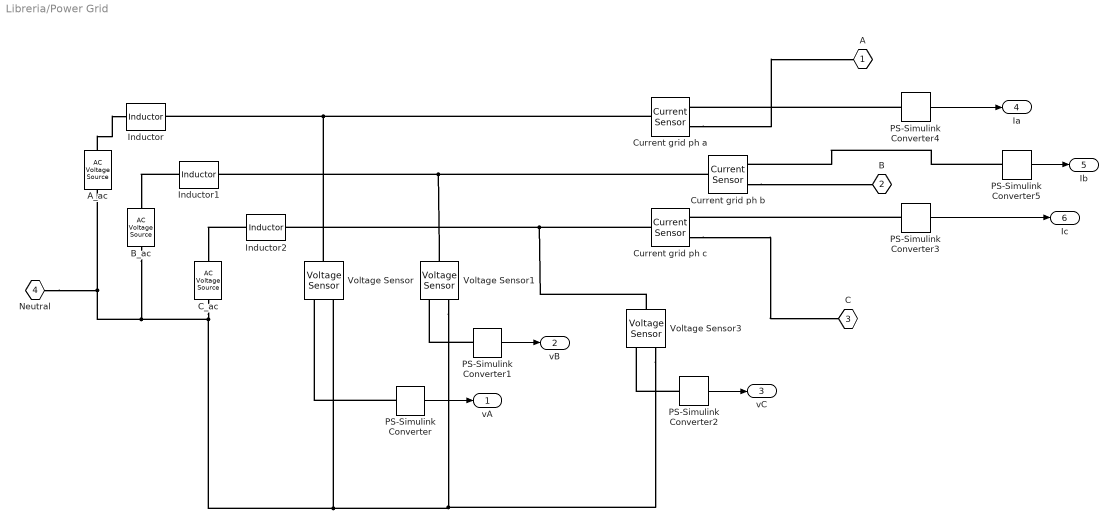
== system Libreria/Power Grid ==
  A_ac : fl_lib/Electrical/Electrical Sources/AC Voltage Source  amp=170 V  shift=0 deg  frequency=60 Hz  omega=0 rad/s
  B_ac : fl_lib/Electrical/Electrical Sources/AC Voltage Source  amp=170 V  shift=-120 deg  frequency=60 Hz  omega=0 rad/s
  C_ac : fl_lib/Electrical/Electrical Sources/AC Voltage Source  amp=170 V  shift=120 deg  frequency=60 Hz  omega=0 rad/s
  Current grid ph a : fl_lib/Electrical/Electrical Sensors/Current Sensor
  Current grid ph b : fl_lib/Electrical/Electrical Sensors/Current Sensor
  Current grid ph c : fl_lib/Electrical/Electrical Sensors/Current Sensor
  Inductor : fl_lib/Electrical/Electrical Elements/Inductor  l=0.1 uH  r=0.2 Ohm  g=1e-9 1/Ohm  i_specify=off  i_priority=None  i=0 A  i_nominal_specify=off  i_nominal_unit=A  i_nominal_value=1  v_specify=off  v_priority=None  v=0 V  v_nominal_specify=off  v_nominal_unit=V  v_nominal_value=1  i_L_specify=on  i_L_priority=High  i_L=0 A  i_L_nominal_specify=off  i_L_nominal_unit=A  i_L_nominal_value=1
  Inductor1 : fl_lib/Electrical/Electrical Elements/Inductor  l=0.1 uH  r=0.2 Ohm  g=1e-9 1/Ohm  i_specify=off  i_priority=None  i=0 A  i_nominal_specify=off  i_nominal_unit=A  i_nominal_value=1  v_specify=off  v_priority=None  v=0 V  v_nominal_specify=off  v_nominal_unit=V  v_nominal_value=1  i_L_specify=on  i_L_priority=High  i_L=0 A  i_L_nominal_specify=off  i_L_nominal_unit=A  i_L_nominal_value=1
  Inductor2 : fl_lib/Electrical/Electrical Elements/Inductor  l=0.1 uH  r=0.2 Ohm  g=1e-9 1/Ohm  i_specify=off  i_priority=None  i=0 A  i_nominal_specify=off  i_nominal_unit=A  i_nominal_value=1  v_specify=off  v_priority=None  v=0 V  v_nominal_specify=off  v_nominal_unit=V  v_nominal_value=1  i_L_specify=on  i_L_priority=High  i_L=0 A  i_L_nominal_specify=off  i_L_nominal_unit=A  i_L_nominal_value=1
  PS-Simulink Converter{,1..5} (6 alike) : nesl_utility/PS-Simulink Converter  PhysicalDomain=network_engine_domain  SubClassName=ps_output  LeftPortType=input  RightPortType=output  PseudoPeriodic=off  Frequencies=[]  Unit=1  AffineConversion=off
  Voltage Sensor : fl_lib/Electrical/Electrical Sensors/Voltage Sensor
  Voltage Sensor1 : fl_lib/Electrical/Electrical Sensors/Voltage Sensor
  Voltage Sensor3 : fl_lib/Electrical/Electrical Sensors/Voltage Sensor
  A : PMIOPort  Port=1  Side=Left
  B : PMIOPort  Port=2  Side=Left
  C : PMIOPort  Port=3  Side=Left
  Neutral : PMIOPort  Port=4  Side=Left
  vA : Outport
  vB : Outport  Port=2
  vC : Outport  Port=3
  Ia : Outport  Port=4
  Ib : Outport  Port=5
  Ic : Outport  Port=6
  wires:
  PS-Simulink Converter/1 -> vA/1
  PS-Simulink Converter1/1 -> vB/1
  PS-Simulink Converter2/1 -> vC/1
  PS-Simulink Converter4/1 -> Ia/1
  PS-Simulink Converter5/1 -> Ib/1
  PS-Simulink Converter3/1 -> Ic/1
  connections:
  Inductor2/LConn1 -- C_ac/LConn1
  A_ac/LConn1 -- Inductor/LConn1
  Inductor1/LConn1 -- B_ac/LConn1
  Voltage Sensor1/LConn1 -- Inductor1/RConn1 -- Current grid ph b/LConn1
  PS-Simulink Converter/LConn1 -- Voltage Sensor/RConn1
  Voltage Sensor3/LConn1 -- Inductor2/RConn1 -- Current grid ph c/LConn1
  Voltage Sensor/LConn1 -- Current grid ph a/LConn1 -- Inductor/RConn1
  A_ac/RConn1 -- Neutral/RConn1 -- Voltage Sensor3/RConn2 -- Voltage Sensor1/RConn2 -- Voltage Sensor/RConn2 -- C_ac/RConn1 -- B_ac/RConn1
  PS-Simulink Converter1/LConn1 -- Voltage Sensor1/RConn1
  PS-Simulink Converter2/LConn1 -- Voltage Sensor3/RConn1
  Current grid ph c/RConn2 -- C/RConn1
  Current grid ph b/RConn2 -- B/RConn1
  Current grid ph a/RConn2 -- A/RConn1
  PS-Simulink Converter3/LConn1 -- Current grid ph c/RConn1
  PS-Simulink Converter4/LConn1 -- Current grid ph a/RConn1
  PS-Simulink Converter5/LConn1 -- Current grid ph b/RConn1

== system Libreria/PowerControlLoop_4CSI ==
  V3 : Inport
  I3 : Inport  Port=2
  P_setpoint : Inport  Port=3
  Q_setpoint : Inport  Port=4
  Alpha_Beta_PRController : Subsystem
      mask Display:
      | port_label('input', 1, 'I_{\alpha ref}', 'texmode', 'on')
      | port_label('input', 2, 'I_{\beta ref}', 'texmode', 'on')
      | port_label('input', 3, '[ I_a, I_b, I_c ]', 'texmode', 'on')
      | 
      | port_label('output', 1, '[ I_{a act}, I_{b act}, I_{c act} ]', 'texmode', 'on')
      | 
      | plot(.65+[0:.01:pi/10], .3+sin(40*[0:.01:pi/10])/13)
      | 
      | %plot([.4 .6],.05+[.5 .7])
      | %plot([.4 .6],.05+[.9 .7])
      | %plot([.4 .4],.05+[.9 .5])
      | 
      | text(.5,.3,'\fontsize{25} \int', 'texmode', 'on')
      | 
      | text(.5,.8,'\fontsize{15} PR_{\alpha \beta}', 'texmode', 'on')
  Demux : Demux  Outputs=3
  Demux1 : Demux  Outputs=3
  Instantaneous p-q transformation : MATLAB Function  TreatAsAtomicUnit=on
  PQ2AlphBetaCurrents : MATLAB Function  TreatAsAtomicUnit=on
  u_a_u_b : Outport
  wires:
  I3/1 -> Alpha_Beta_PRController/3(I3), Demux1/1
  PQ2AlphBetaCurrents/1(Ia) -> Alpha_Beta_PRController/1(Ia_ref)
  V3/1 -> Demux/1
  Alpha_Beta_PRController/1(Iab_act) -> u_a_u_b/1
  Demux/1 -> Instantaneous p-q transformation/1(va)
  Demux1/3 -> Instantaneous p-q transformation/6(ic)
  Demux1/1 -> Instantaneous p-q transformation/4(ia)
  Demux1/2 -> Instantaneous p-q transformation/5(ib)
  P_setpoint/1 -> PQ2AlphBetaCurrents/3(p)
  Q_setpoint/1 -> PQ2AlphBetaCurrents/4(q)
  PQ2AlphBetaCurrents/2(Ib) -> Alpha_Beta_PRController/2(ib_ref)
  Demux/3 -> Instantaneous p-q transformation/3(vc)
  Instantaneous p-q transformation/9(ValA) -> PQ2AlphBetaCurrents/1(Va)
  Instantaneous p-q transformation/10(VbetA) -> PQ2AlphBetaCurrents/2(Vb)
  Demux/2 -> Instantaneous p-q transformation/2(vb)

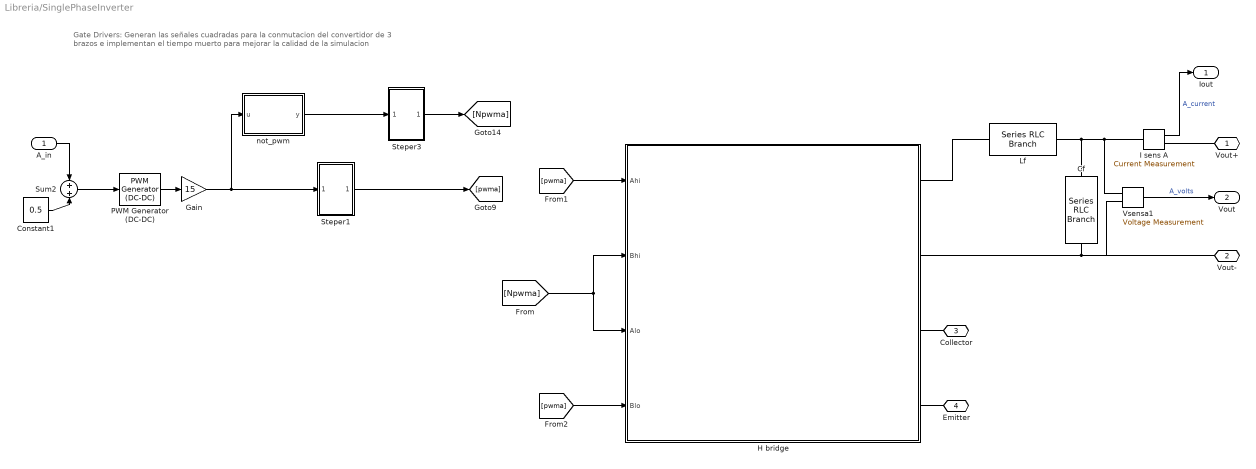
== system Libreria/SinglePhaseInverter ==
  note: Gate Drivers: Generan las señales cuadradas para
      | la conmutacion del convertidor de 3 brazos e implementan el
      | tiempo muerto para mejorar la calidad de la simulacion
  A_in : Inport
  Cf : powerlib/Elements/Series RLC Branch  LConnTagsString=__new0  RConnTagsString=__new0  BranchType=C  Resistance=1  Inductance=1e-3  SetiL0=off  InitialCurrent=0  Capacitance=2.2e-6  Setx0=off  InitialVoltage=0  Measurements=None
  Constant1 : Constant  Value=0.5
  Gain : Gain  Gain=15
  H bridge : Subsystem
      mask Display:
      | port_label('input', 1, '\fontsize{12} Ahi', 'texmode', 'on')
      | port_label('input', 2, '\fontsize{12} Alo', 'texmode', 'on')
      | port_label('input', 3, '\fontsize{12} Bhi', 'texmode', 'on')
      | port_label('input', 4, '\fontsize{12} Blo', 'texmode', 'on')
      | 
      | 
      | port_label('rconn', 1, '\fontsize{12} V_{out} +', 'texmode', 'on')
      | port_label('rconn', 2, '\fontsize{12} V_{out} -', 'texmode', 'on')
      | 
      | port_label('rconn', 3, '\fontsize{12} Collector', 'texmode', 'on')
      | port_label('rconn', 4, '\fontsize{12} Emitter', 'texmode', 'on')
      | 
      | lvx = [.1 .1];
      | lvy = [.1 .2];
      | lhx = [.1 .2];
      | lhy = [.1 .1];
      | 
      | 
      | % se dibujan los interruptores de la izquierda
      | plot(lvx+.07, lvy*.8+.028+.1)
      | plot(lvx+.1, lvy+.1)
      | plot(lhx*.5+.15, lhy+.1)
      | plot(lhx*.5+.15, lhy+.2)
      | plot(lhx*.5+.07, lhy+.15)
      | 
      | d=0.5;
      | 
      | plot(lvx+.07, lvy*.8+.028+.1+d)
      | plot(lvx+.1, lvy+.1+d)
      | plot(lhx*.5+.15, lhy+.1+d)
      | plot(lhx*.5+.15, lhy+.2+d)
      | plot(lhx*.5+.07, lhy+.15+d)
      | 
      | 
      | % se dibujan los interruptores del medio
      | h=.3;
      | 
      | %plot(lvx+.07+h, lvy*.8+.028+.1)
      | %plot(lvx+.1+h, lvy+.1)
      | %plot(lhx*.5+.15+h, lhy+.1)
      | %plot(lhx*.5+.15+h, lhy+.2)
      | %plot(lhx*.5+.07+h, lhy+.15)
      | 
      | %plot(lvx+.07+h, lvy*.8+.028+.1+d)
      | %plot(lvx+.1+h, lvy+.1+d)
      | %plot(lhx*.5+.15+h, lhy+.1+d)
      | %plot(lhx*.5+.15+h, lhy+.2+d)
      | %plot(lhx*.5+.07+h, lhy+.15+d)
      | 
      | % se dibujan los interruptores de la derecha
      | h=.6
      | 
      | plot(lvx+.07+h, lvy*.8+.028+.1)
      | plot(lvx+.1+h, lvy+.1)
      | plot(lhx*.5+.15+h, lhy+.1)
      | plot(lhx*.5+.15+h, lhy+.2)
      | plot(lhx*.5+.07+h, lhy+.15)
      | 
      | plot(lvx+.07+h, lvy*.8+.028+.1+d)
      | plot(lvx+.1+h, lvy+.1+d)
      | plot(lhx*.5+.15+h, lhy+.1+d)
      | plot(lhx*.5+.15+h, lhy+.2+d)
      | plot(lhx*.5+.07+h, lhy+.15+d)
      | 
      | 
      | % se conectan los interruptores.
      | plot(lvx+.15, lvy*4-.1)
      | %plot(lvx+.15+.3, lvy*4-.1)
      | plot(lvx+.15+.6, lvy*4-.1)
      | 
      | 
      | plot(lvx+.15, lvy+.7)
      | %plot(lvx+.15+.3, lvy+.7)
      | plot(lvx+.15+.6, lvy+.7)
      | 
      | plot(lvx+.15, lvy)
      | %plot(lvx+.15+.3, lvy)
      | plot(lvx+.15+.6, lvy)
      | 
      | plot(lhx*6-.35, lhy)
      | plot(lhx*6-.35, lhy+.8)
      | 
      | % raul esteban alzate 313 515 86 11
  I sens A : powerlib/Measurements/Current Measurement  PhasorSimulation=off  OutputType=Complex  PSBequivalent=0
  Lf : powerlib/Elements/Series RLC Branch  LConnTagsString=__new0  RConnTagsString=__new0  BranchType=RL  Resistance=.1  Inductance=10e-3  SetiL0=off  InitialCurrent=0  Capacitance=1e-6  Setx0=off  InitialVoltage=0  Measurements=None
  PWM Generator (DC-DC) : powerlib_meascontrol/Pulse & Signal Generators/PWM Generator (DC-DC)  Fsw=f_sw  Ts=0
  Steper1 : Subsystem
  Steper3 : Subsystem
  Sum2 : Sum
  Vsensa1 : powerlib/Measurements/Voltage Measurement  PhasorSimulation=off  OutputType=Complex  PSBequivalent=0
  not_pwm : MATLAB Function  TreatAsAtomicUnit=on
  Vout+ : PMIOPort  Port=1  Side=Right
  Vout- : PMIOPort  Port=2  Side=Right
  Collector : PMIOPort  Port=3  Side=Left
  Emitter : PMIOPort  Port=4  Side=Left
  Iout : Outport
  Vout : Outport  Port=2
  wires:
  not_pwm/1(y) -> Steper3/1(In1)
  Sum2/1 -> PWM Generator (DC-DC)/1
  PWM Generator (DC-DC)/1 -> Gain/1
  Constant1/1 -> Sum2/2
  A_in/1 -> Sum2/1
  Steper1/1(Out1) -> [pwma]
  Steper3/1(Out1) -> [Npwma]
  Gain/1 -> Steper1/1(In1), not_pwm/1(u)
  [pwma] -> H bridge/1(Ahi)
  [Npwma] -> H bridge/2(Bhi), H bridge/3(Alo)
  [pwma] -> H bridge/4(Blo)
  I sens A/1 -> Iout/1  "A_current"
  Vsensa1/1 -> Vout/1  "A_volts"
  connections:
  H bridge/RConn3 -- Collector/RConn1
  H bridge/RConn4 -- Emitter/RConn1
  Lf/LConn1 -- H bridge/RConn1
  I sens A/LConn1 -- Cf/LConn1 -- Lf/RConn1 -- Vsensa1/LConn1
  H bridge/RConn2 -- Vout-/RConn1 -- Vsensa1/LConn2 -- Cf/RConn1
  Vout+/RConn1 -- I sens A/RConn1

== system Libreria/Alpha_Beta_PRController/PR Controller_0_ref 1 ==
  ref : Inport
  real : Inport  Port=2
  K1 : Gain  Gain=2/100
  K2 : Gain  Gain=10
  Steper6 : Subsystem
  Sum : Sum  Inputs=+-
  Sum1 : Sum  Inputs=+|+
  Transfer Fcn : TransferFcn  Numerator=[1 0]  Denominator=[1 20 (60*2*pi)^2]
  Out1 : Outport
  wires:
  Sum1/1 -> Out1/1
  Steper6/1(Out1) -> K2/1, K1/1
  K2/1 -> Transfer Fcn/1
  Transfer Fcn/1 -> Sum1/2
  K1/1 -> Sum1/1
  Sum/1 -> Steper6/1(In1)
  ref/1 -> Sum/1
  real/1 -> Sum/2

== system Libreria/Alpha_Beta_PRController/PR Controller_0_ref 3 ==
  ref : Inport
  real : Inport  Port=2
  K1 : Gain  Gain=2/100
  K2 : Gain  Gain=10
  Steper6 : Subsystem
  Sum : Sum  Inputs=+-
  Sum1 : Sum  Inputs=+|+
  Transfer Fcn : TransferFcn  Numerator=[1 0]  Denominator=[1 20 (60*2*pi)^2]
  Out1 : Outport
  wires:
  real/1 -> Sum/2
  ref/1 -> Sum/1
  Sum/1 -> Steper6/1(In1)
  K1/1 -> Sum1/1
  Transfer Fcn/1 -> Sum1/2
  K2/1 -> Transfer Fcn/1
  Steper6/1(Out1) -> K1/1, K2/1
  Sum1/1 -> Out1/1

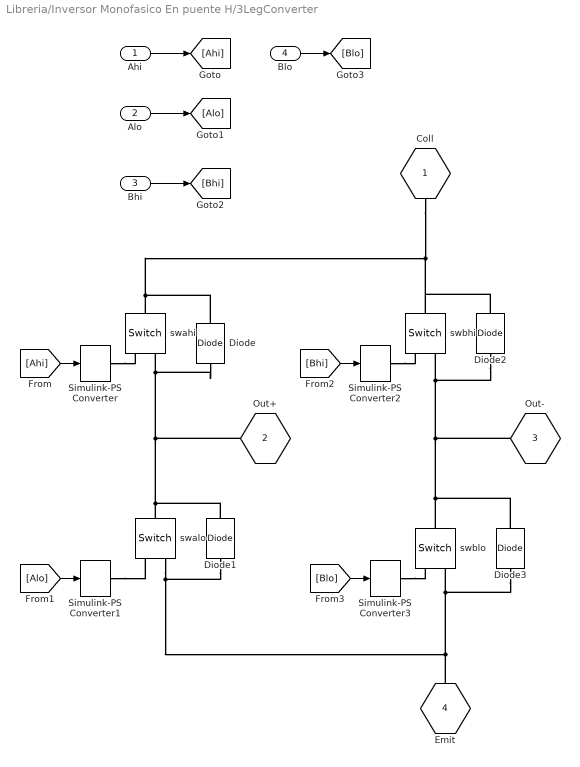
== system Libreria/Inversor Monofasico En puente H/3LegConverter ==
  Ahi : Inport
  Alo : Inport  Port=2
  Bhi : Inport  Port=3
  Blo : Inport  Port=4
  Diode{,1..3} (4 alike) : fl_lib/Electrical/Electrical Elements/Diode  Vf=0.6 V  Ron=0.3 Ohm  Goff=1e-8 1/Ohm  i_specify=off  i_priority=None  i=0 A  i_nominal_specify=off  i_nominal_unit=A  i_nominal_value=1  v_specify=off  v_priority=None  v=0 V  v_nominal_specify=off  v_nominal_unit=V  v_nominal_value=1
  Simulink-PS Converter{,1..3} (4 alike) : nesl_utility/Simulink-PS Converter  PhysicalDomain=network_engine_domain  SubClassName=ps_input  LeftPortType=input  RightPortType=output  PseudoPeriodic=off  Frequencies=[]  NoiseDistribution=none  NoiseParameters=[]  Unit=1  AffineConversion=off  FilteringAndDerivatives=zero  SimscapeFilterOrder=1  InputFilterTimeConstant=0.001  UdotUserProvided=1
  swahi : fl_lib/Electrical/Electrical Elements/Switch  R_closed=0.01 Ohm  G_open=1e-8 1/Ohm  Threshold=2  i_specify=off  i_priority=None  i=0 A  i_nominal_specify=off  i_nominal_unit=A  i_nominal_value=1  v_specify=off  v_priority=None  v=0 V  v_nominal_specify=off  v_nominal_unit=V  v_nominal_value=1
      settings: SourceProductName=Simscape
  swalo : fl_lib/Electrical/Electrical Elements/Switch  R_closed=0.01 Ohm  G_open=1e-8 1/Ohm  Threshold=2  i_specify=off  i_priority=None  i=0 A  i_nominal_specify=off  i_nominal_unit=A  i_nominal_value=1  v_specify=off  v_priority=None  v=0 V  v_nominal_specify=off  v_nominal_unit=V  v_nominal_value=1
      settings: SourceProductName=Simscape
  swbhi : fl_lib/Electrical/Electrical Elements/Switch  R_closed=0.01 Ohm  G_open=1e-8 1/Ohm  Threshold=2  i_specify=off  i_priority=None  i=0 A  i_nominal_specify=off  i_nominal_unit=A  i_nominal_value=1  v_specify=off  v_priority=None  v=0 V  v_nominal_specify=off  v_nominal_unit=V  v_nominal_value=1
      settings: SourceProductName=Simscape
  swblo : fl_lib/Electrical/Electrical Elements/Switch  R_closed=0.01 Ohm  G_open=1e-8 1/Ohm  Threshold=2  i_specify=off  i_priority=None  i=0 A  i_nominal_specify=off  i_nominal_unit=A  i_nominal_value=1  v_specify=off  v_priority=None  v=0 V  v_nominal_specify=off  v_nominal_unit=V  v_nominal_value=1
      settings: SourceProductName=Simscape
  Coll : PMIOPort  Port=1  Side=Right
  Out+ : PMIOPort  Port=2  Side=Right
  Out- : PMIOPort  Port=3  Side=Right
  Emit : PMIOPort  Port=4  Side=Right
  wires:
  [Alo] -> Simulink-PS Converter1/1
  [Ahi] -> Simulink-PS Converter/1
  Alo/1 -> [Alo]
  [Blo] -> Simulink-PS Converter3/1
  Bhi/1 -> [Bhi]
  [Bhi] -> Simulink-PS Converter2/1
  Ahi/1 -> [Ahi]
  Blo/1 -> [Blo]
  connections:
  swalo/RConn2 -- Diode3/LConn1 -- swblo/RConn2 -- Emit/RConn1 -- Diode1/LConn1
  Simulink-PS Converter/RConn1 -- swahi/RConn1
  swblo/LConn1 -- Diode3/RConn1 -- Out-/RConn1 -- Diode2/LConn1 -- swbhi/RConn2
  Simulink-PS Converter3/RConn1 -- swblo/RConn1
  Simulink-PS Converter2/RConn1 -- swbhi/RConn1
  Simulink-PS Converter1/RConn1 -- swalo/RConn1
  swalo/LConn1 -- Out+/RConn1 -- Diode/LConn1 -- swahi/RConn2 -- Diode1/RConn1
  swahi/LConn1 -- Diode/RConn1 -- Coll/RConn1 -- Diode2/RConn1 -- swbhi/LConn1

== system Libreria/Inversor Monofasico En puente H/Isens2 ==
  Current Sensor : fl_lib/Electrical/Electrical Sensors/Current Sensor
  PS-Simulink Converter : nesl_utility/PS-Simulink Converter  PhysicalDomain=network_engine_domain  SubClassName=ps_output  LeftPortType=input  RightPortType=output  PseudoPeriodic=off  Frequencies=[]  Unit=1  AffineConversion=off
  + : PMIOPort  Port=1  Side=Left
  - : PMIOPort  Port=2  Side=Right
  i : Outport
  wires:
  PS-Simulink Converter/1 -> i/1
  connections:
  PS-Simulink Converter/LConn1 -- Current Sensor/RConn1
  Current Sensor/RConn2 -- -/RConn1
  Current Sensor/LConn1 -- +/RConn1

== system Libreria/Inversor Monofasico En puente H/Steper1 ==
  In1 : Inport
  Product : Product
  Step : Step  Time=st_time3  SampleTime=0
  Out1 : Outport
  wires:
  Step/1 -> Product/2
  In1/1 -> Product/1
  Product/1 -> Out1/1

== system Libreria/Inversor Monofasico En puente H/Steper3 ==
  In1 : Inport
  Product : Product
  Step : Step  Time=st_time3  SampleTime=0
  Out1 : Outport
  wires:
  Product/1 -> Out1/1
  In1/1 -> Product/1
  Step/1 -> Product/2
